simulink model "SEA_modelPOG"  (Simulink 7.2)
settings: Solver=ode45  StartTime=0.0  StopTime=10.0  RelTol=1e-3
values from neighbouring files (symbols this model uses):
  g = 9.81    [TSC150918ProvaMatlab.m]
  l = 0.5    [TSC150918ProvaMatlab.m]
undefined symbols (not defined in the file or in its folder): B, D, I, K, M, T
settings Model: Creator=lbiagiotti  LastModifiedBy=lbiagiotti

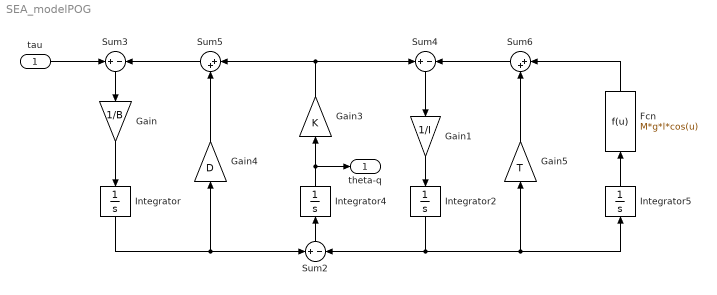
== system SEA_modelPOG ==
  tau : Inport  OutDataType=sfix(16)  OutScaling=2^0
  Fcn : Fcn  Orientation=up  Expr=M*g*l*cos(u)
  Gain : Gain  Orientation=down  Gain=1/B  ParameterDataType=sfix(16)  ParameterScaling=2^0  OutDataType=sfix(16)  OutScaling=2^0
  Gain1 : Gain  Orientation=down  Gain=1/I  ParameterDataType=sfix(16)  ParameterScaling=2^0  OutDataType=sfix(16)  OutScaling=2^0
  Gain3 : Gain  Orientation=up  Gain=K  ParameterDataType=sfix(16)  ParameterScaling=2^0  OutDataType=sfix(16)  OutScaling=2^0
  Gain4 : Gain  Orientation=up  Gain=D  ParameterDataType=sfix(16)  ParameterScaling=2^0  OutDataType=sfix(16)  OutScaling=2^0
  Gain5 : Gain  Orientation=up  Gain=T  ParameterDataType=sfix(16)  ParameterScaling=2^0  OutDataType=sfix(16)  OutScaling=2^0
  Integrator : Integrator  Orientation=down
  Integrator2 : Integrator  Orientation=down
  Integrator4 : Integrator  Orientation=up
  Integrator5 : Integrator  Orientation=up
  Sum2 : Sum  Orientation=up  Inputs=+-  OutDataType=sfix(16)  OutScaling=2^0
  Sum3 : Sum  Orientation=down  Inputs=+-  OutDataType=sfix(16)  OutScaling=2^0
  Sum4 : Sum  Orientation=down  Inputs=+-  OutDataType=sfix(16)  OutScaling=2^0
  Sum5 : Sum  Orientation=left  Inputs=|++  OutDataType=sfix(16)  OutScaling=2^0
  Sum6 : Sum  Orientation=left  Inputs=|++  OutDataType=sfix(16)  OutScaling=2^0
  theta-q : Outport  OutDataType=sfix(16)  OutScaling=2^0
  wires:
  Gain/1 -> Integrator/1
  Gain1/1 -> Integrator2/1
  Integrator/1 -> Sum2/1, Gain4/1
  Sum2/1 -> Integrator4/1
  Integrator4/1 -> Gain3/1, theta-q/1
  Sum3/1 -> Gain/1
  Gain3/1 -> Sum4/1, Sum5/1
  Sum4/1 -> Gain1/1
  tau/1 -> Sum3/1
  Gain4/1 -> Sum5/2
  Sum5/1 -> Sum3/2
  Integrator2/1 -> Gain5/1, Integrator5/1, Sum2/2
  Gain5/1 -> Sum6/2
  Sum6/1 -> Sum4/2
  Fcn/1 -> Sum6/1
  Integrator5/1 -> Fcn/1
